simulink library "lib_GenTools_MinMax"  (R2015a)
settings: Solver=ode45  StartTime=0.0  StopTime=10.0  RelTol=1e-3
settings Model: Creator=jlkratz  LastModifiedBy=jlkratz

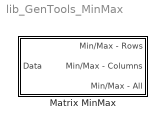
== system lib_GenTools_MinMax ==
  Matrix MinMax : Subsystem  mask(TSAT: Matrix MinMax Block){rows_M=on, cols_M=on, all_M=on, minmax_M=off, BN_M=gcb}
      mask prompts: rows_M "rows_M - Min/Max of Rows"; cols_M "cols_M - Min/Max ofColumns"; all_M "all_M - Min/Max of  All"; minmax_M "minmax_M - checked for min and unchecked for max"; BN_M "BN_M - Block Name"
      mask help: This block is meant for determining the minimum and maximum value(s) in 1-D and 2-D arrays. It can be used to return the min or max of the rows, columns, or all values within the data set.
      mask init:
      | % Setup Outports ---------------------------------------------------------%
      | 
      | % Outport Numbers
      | n = 1; %first inport
      | 
      | % Average Rows Inport
      | if rows_M == 1
      |     if strcmp(get_param([BN_M '/Min//Max - Rows'],'BlockType'),'Terminator')
      |         MSK_ReplaceBlock_TSAT([BN_M '/Min//Max - Rows'],'built-in/Outport');
      |     end
      |     set_param([BN_M '/Min//Max - Rows'],'Port',num2str(n));
      |     n = n + 1;
      | elseif rows_M == 0
      |     if strcmp(get_param([BN_M '/Min//Max - Rows'],'BlockType'),'Outport')
      |         MSK_ReplaceBlock_TSAT([BN_M '/Min//Max - Rows'],'built-in/Terminator');
      |     end
      | end
      | 
      | % Average Columns Inport
      | if cols_M == 1
      |     if strcmp(get_param([BN_M '/Min//Max - Columns'],'BlockType'),'Terminator')
      |         MSK_ReplaceBlock_TSAT([BN_M '/Min//Max - Columns'],'built-in/Outport');
      |     end
      |     set_param([BN_M '/Min//Max - Columns'],'Port',num2str(n));
      |     n = n + 1;
      | elseif cols_M == 0
      |     if strcmp(get_param([BN_M '/Min//Max - Columns'],'BlockType'),'Outport')
      |         MSK_ReplaceBlock_TSAT([BN_M '/Min//Max - Columns'],'built-in/Terminator');
      |     end
      | end
      | 
      | % Average All Inport
      | if all_M == 1
      |     if strcmp(get_param([BN_M '/Min//Max - All'],'BlockType'),'Terminator')
      |         MSK_ReplaceBlock_TSAT([BN_M '/Min//Max - All'],'built-in/Outport');
      |     end
      |     set_param([BN_M '/Min//Max - All'],'Port',num2str(n));
      |     n = n + 1;
      | elseif all_M == 0
      |     if strcmp(get_param([BN_M '/Min//Max - All'],'BlockType'),'Outport')
      |         MSK_ReplaceBlock_TSAT([BN_M '/Min//Max - All'],'built-in/Terminator');
      |     end
      | end
      mask Help: web(which('GenTools_TSAT_MinMax.html'),'-helpbrowser')

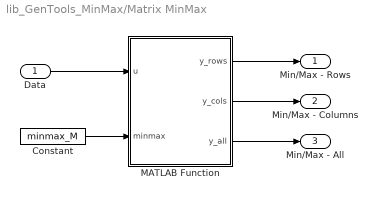
== system lib_GenTools_MinMax/Matrix MinMax ==
  Data : Inport
  Constant : Constant  Value=minmax_M
  MATLAB Function : MATLAB Function  TreatAsAtomicUnit=on
  Min/Max - Rows : Outport
  Min/Max - Columns : Outport  Port=2
  Min/Max - All : Outport  Port=3
  wires:
  MATLAB Function/3(y_all) -> Min/Max - All/1
  MATLAB Function/2(y_cols) -> Min/Max - Columns/1
  MATLAB Function/1(y_rows) -> Min/Max - Rows/1
  Data/1 -> MATLAB Function/1(u)
  Constant/1 -> MATLAB Function/2(minmax)

== matlab function lib_GenTools_MinMax/Matrix MinMax/MATLAB Function ==
  data: u input; y_rows output; y_cols output; y_all output; minmax input
function [y_rows, y_cols, y_all] = minmax_mat(u,minmax)
%#codegen

[n,m] = size(u);

%min/max rows
y_rows = zeros(n,1);
for i = 1:n
    if minmax == 1
        y_rows(i) = min(u(i,:));
    else
        y_rows(i) = max(u(i,:));
    end
end

%min/max columns
y_cols = zeros(1,m);
for j = 1:m
    if minmax == 1
        y_cols(j) = min(u(:,j));
    else
        y_cols(j) = max(u(:,j));
    end
end
    
%min/max all   
if minmax == 1
    y_all = min(min(u));
else
    y_all = max(max(u));
end
